simulink model "zbiornik_sys"  (R2024b)
settings: Solver=VariableStepAuto  StartTime=0.0  StopTime=10.0  RelTol=1e-3
settings Model: Creator=mati  LastModifiedBy=mati

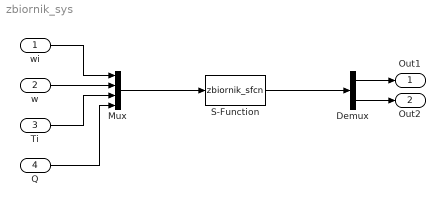
== system zbiornik_sys ==
  wi : Inport
  w : Inport  Port=2
  Ti : Inport  Port=3
  Q : Inport  Port=4
  Demux : Demux  Outputs=2
  Mux : Mux
  S-Function : S-Function  FunctionName=zbiornik_sfcn  Parameters=V_0 T_0  SFunctionDeploymentMode=off  EnableBusSupport=off
  Out1 : Outport  SignalName=V
  Out2 : Outport  Port=2  SignalName=T
  wires:
  wi/1 -> Mux/1
  w/1 -> Mux/2
  Ti/1 -> Mux/3
  Q/1 -> Mux/4
  Mux/1 -> S-Function/1
  S-Function/1 -> Demux/1
  Demux/1 -> Out1/1
  Demux/2 -> Out2/1
